simulink subsystem "PieroAJ"  (R2023b)
settings: Solver=VariableStepAuto  StartTime=0.0  StopTime=10.0  RelTol=1e-3
settings Model: Creator=USUARIO  LastModifiedBy=USUARIO

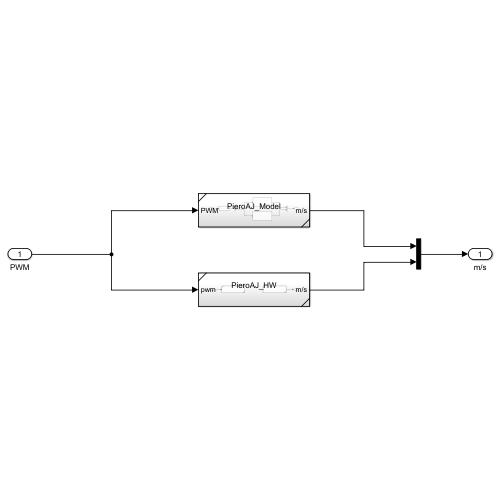
[thumbnail: Simulink's stored preview of the top-level diagram]
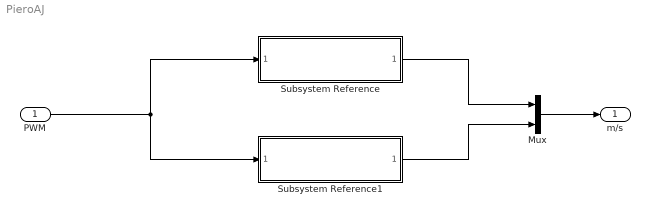
== system PieroAJ ==
  PWM : Inport
  Mux : Mux  Inputs=2
  Subsystem Reference : Subsystem  ReferencedSubsystem=PieroAJ_Model
  Subsystem Reference1 : Subsystem  ReferencedSubsystem=PieroAJ_HW
  m/s : Outport
  wires:
  PWM/1 -> Subsystem Reference1/1, Subsystem Reference/1
  Mux/1 -> m/s/1
  Subsystem Reference1/1 -> Mux/2
  Subsystem Reference/1 -> Mux/1
